simulink model "traj_test_gen"  (R2023a)
settings: Solver=ode1  StartTime=0.0  StopTime=500  FixedStep=Ts  RelTol=1e-3
libraries: shareduavrstlib x1
settings Model: Creator=stt  LastModifiedBy=stt

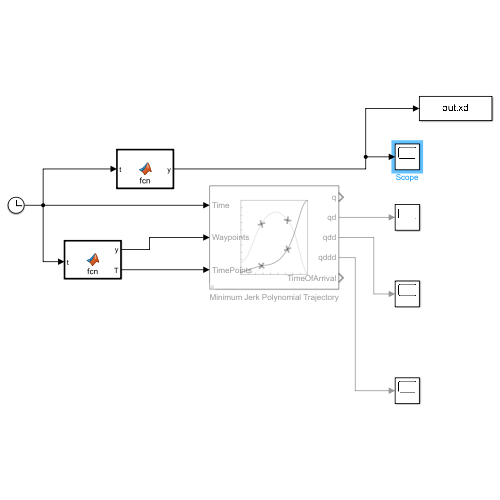
[thumbnail: Simulink's stored preview of the top-level diagram]
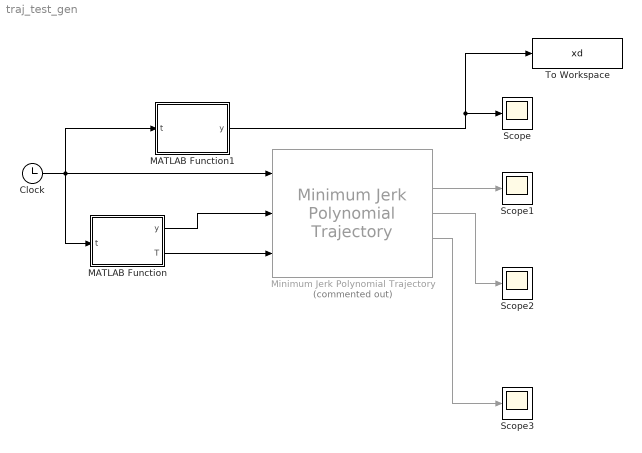
== system traj_test_gen ==
  Clock : Clock
  MATLAB Function : MATLAB Function  TreatAsAtomicUnit=on
  MATLAB Function1 : MATLAB Function  TreatAsAtomicUnit=on
  Minimum Jerk Polynomial Trajectory : shareduavrstlib/Minimum Jerk Polynomial Trajectory  Commented=on  ShowBCInputPort=off  ShowPolynomialCoefs=off  ShowStatusOutputPort=off  TimeAllocation=off  TimeWeight=100  MinSegmentTime=0.1  MaxSegmentTime=1  MaxIteration=1500  MaxTime=10  SimulateUsing=Interpreted execution
      settings: LibrarySourceBlock=robotutilslib/Minimum Jerk Polynomial Trajectory
  Scope{,1..3} (4 alike) : Scope
  To Workspace : ToWorkspace  VariableName=xd  SaveFormat=Timeseries  SampleTime=-1
  wires:
  MATLAB Function/1(y) -> Minimum Jerk Polynomial Trajectory/2
  MATLAB Function/2(T) -> Minimum Jerk Polynomial Trajectory/3
  Clock/1 -> MATLAB Function/1(t), MATLAB Function1/1(t), Minimum Jerk Polynomial Trajectory/1
  MATLAB Function1/1(y) -> To Workspace/1, Scope/1
  Minimum Jerk Polynomial Trajectory/2 -> Scope1/1
  Minimum Jerk Polynomial Trajectory/3 -> Scope2/1
  Minimum Jerk Polynomial Trajectory/4 -> Scope3/1

== matlab function traj_test_gen/MATLAB Function ==
  data: y output; T output; t input
function [y,T] = fcn(t)

T0=300:20:400;
% y1=[0 1.8824    1.8287   -0.0585    1.2011   -1.4325   -0.3130    1.6629    1.1688    1.8380    0.6230   -1.8572...
%     1.3965    1.7360    0.7149    1.0310    0.9725   -0.4311    0.6219   -1.3153    0.8242   -1.8727];
% y2=[-0.7316
%     -1.8622
%    -0.2450
%    0]';

% y=[0, 0.9442    1.2174   -1.1190    1.2401    0.3971   -1.2074   -0.6645    0.1406    1.3725    1.3947   -1.0272...
%     1.4118    1.3715   -0.0439    0.9008   -1.0743   -0.2347    1.2472    0.8766    1.3785    0.4672   -1.3929...
% 1.0474      0.7732 0]/1.5;
% y=[0,  -0.0439    0.9008   -1.0743   -0.2347    1.2472    0.8766    1.3785    0.4672   -1.3929...
% 1.0474      0.7732 0];
if t<300
    T=linspace(1,300,length(T0));
    y=-0.5*ones(1,length(T));
else
    T=T0;
    y=[-0.5, -0.3897    -0.6469     -0.1225    -0.3658  -0.5];
    % y=1.5*[0, 0.6469    0.3897   -0.3658    0.9004   -0.9311   -0.1225   -0.2369    0.5310    0.5904,0];
end

== matlab function traj_test_gen/MATLAB Function1 ==
  data: y output; t input
function y = fcn(t)

T=25;

if t<300
    
    y=-0.3;
elseif t<400
    y=-0.3+0.15*sin((t-300)*2*pi/T);
else
    y=-0.3;
end
